simulink model "Model_TranslationEngine64"  (R2022b)
settings: Solver=FixedStepDiscrete  StartTime=0.0  StopTime=5  RelTol=1e-3  EnableMultiTasking=on
InitFcn:
  | % Initialize model
  | ModelSettings=BTConfig.GetModelSettings();
  | 
  | ModelSettings.Validate();
  | 
  | ModelInit;
  | 
  | 
  | % load library data
  | GainLibrary_data;
  | % Load saved values from partition process
  | CapturedConstMask.LoadMapFromFile(bdroot)
StartFcn:
  | % make sure all the simulated RTC requests are found
  | %RTC_SIM_OBJ.ValidateREQs();
undefined symbols (not defined in the file or in its folder): AA, BPLP, Column, NumHFRefBPF, NumHFRefLPF, NumMusicChannels, Row, VolumeMuteConfig
libraries: TuneVar x925, TOP x490, FeaturePath x111, CapturedConstLib x52
(part 15 of 34)

== system Model_TranslationEngine64/NEAR/Near1p1/VolumeMute/AnnouncementLevelDetector/ch2_level/hold_margin ==
  SetPositive : MATLAB Function  TreatAsAtomicUnit=on
  TOP : TOP/TOP  TriggerInit=[440 20 640 80]  TopName=HoldMarginDb  DataTypeOut=Inherit: Same as input  BankNumber=0  PreOverlay=false  PostOverlay=false  Role=Automatic
      settings: SourceProductName=Bose Talaria
  TranslateTrigger : TuneVar/TranslateTrigger  TriggerInit=[306 -100 344 -45]
      settings: SourceProductName=Bose Talaria
  Tune Variable : TuneVar/TuneVar  TuneName=HoldMarginDb  SpecifyMaxSize=off  VariableDim=1 (Row)  MaxSize=[1 1]  TunabilityNumber=1  MinValue=[]  MaxValue=[]  TriggerInit=[-120 22 90 78]  MaskValue=Config.DefaultAnn2LevelDetectHoldMarginDb
      settings: SourceProductName=Bose Talaria
  wires:
  TranslateTrigger/1 -> SetPositive/Trigger
  SetPositive/1(TOP) -> TOP/1
  Tune Variable/1 -> SetPositive/1(Tune)  "HoldMarginDb"

== system Model_TranslationEngine64/NEAR/Near1p1/VolumeMute/AnnouncementLevelDetector/ch2_level/hold_time ==
  TOP : TOP/TOP  TriggerInit=[475 15 725 85]  TopName=HoldTimeSamples  DataTypeOut=Inherit: Same as input  BankNumber=0  PreOverlay=false  PostOverlay=false  Role=Automatic
      settings: SourceProductName=Bose Talaria
  TranslateTrigger : TuneVar/TranslateTrigger  TriggerInit=[306 -100 344 -45]
      settings: SourceProductName=Bose Talaria
  Tune Variable : TuneVar/TuneVar  TuneName=HoldTimes  SpecifyMaxSize=off  VariableDim=1 (Row)  MaxSize=[1 1]  TunabilityNumber=1  MinValue=[]  MaxValue=[]  TriggerInit=[-100 15 150 85]  MaskValue=Config.DefaultAnn2LevelDetectHoldTimes
      settings: SourceProductName=Bose Talaria
  sec2samples : MATLAB Function  TreatAsAtomicUnit=on  mask{FrameRate=Config.FrameRate}
  wires:
  TranslateTrigger/1 -> sec2samples/Trigger
  sec2samples/1(y) -> TOP/1
  Tune Variable/1 -> sec2samples/1(u)  "HoldTimes"

== system Model_TranslationEngine64/NEAR/Near1p1/VolumeMute/AnnouncementLevelDetector/ch2_level/max_volume ==
  TOP : TOP/TOP  TriggerInit=[440 20 585 80]  TopName=MaxVolumeDb  DataTypeOut=single  BankNumber=BankNumber  PreOverlay=PreOverlay  PostOverlay=PostOverlay  Role=Automatic
      settings: SourceProductName=Bose Talaria
  TrivialTranslation : TuneVar/TrivialTranslation  TriggerInit=[300 28 350 72]
      settings: SourceProductName=Bose Talaria
  Tune Variable : TuneVar/TuneVar  TuneName=MaxVolumeDb  SpecifyMaxSize=off  VariableDim=1 (Row)  MaxSize=[1 1]  TunabilityNumber=1  MinValue=MinValue  MaxValue=MaxValue  TriggerInit=[20 25 190 75]  MaskValue=MaskValue
      settings: SourceProductName=Bose Talaria
  wires:
  Tune Variable/1 -> TrivialTranslation/1  "MaxVolumeDb"
  TrivialTranslation/1 -> TOP/1

== system Model_TranslationEngine64/NEAR/Near1p1/VolumeMute/AnnouncementLevelDetector/ch2_level/min_volume ==
  TOP : TOP/TOP  TriggerInit=[440 20 585 80]  TopName=MinVolumeDb  DataTypeOut=single  BankNumber=BankNumber  PreOverlay=PreOverlay  PostOverlay=PostOverlay  Role=Automatic
      settings: SourceProductName=Bose Talaria
  TrivialTranslation : TuneVar/TrivialTranslation  TriggerInit=[300 28 350 72]
      settings: SourceProductName=Bose Talaria
  Tune Variable : TuneVar/TuneVar  TuneName=MinVolumeDb  SpecifyMaxSize=off  VariableDim=1 (Row)  MaxSize=[1 1]  TunabilityNumber=1  MinValue=MinValue  MaxValue=MaxValue  TriggerInit=[20 25 190 75]  MaskValue=MaskValue
      settings: SourceProductName=Bose Talaria
  wires:
  Tune Variable/1 -> TrivialTranslation/1  "MinVolumeDb"
  TrivialTranslation/1 -> TOP/1

== system Model_TranslationEngine64/NEAR/Near1p1/VolumeMute/AnnouncementLevelDetector/ch2_level/slow_decay ==
  TOP : TOP/TOP  TriggerInit=[440 17 695 83]  TopName=SlowDecayDbPerSample  DataTypeOut=Inherit: Same as input  BankNumber=0  PreOverlay=false  PostOverlay=false  Role=Automatic
      settings: SourceProductName=Bose Talaria
  TranslateTrigger : TuneVar/TranslateTrigger  TriggerInit=[306 -100 344 -45]
      settings: SourceProductName=Bose Talaria
  Tune Variable : TuneVar/TuneVar  TuneName=SlowDecayDbPers  SpecifyMaxSize=off  VariableDim=1 (Row)  MaxSize=[1 1]  TunabilityNumber=1  MinValue=[]  MaxValue=[]  TriggerInit=[-100 17 155 83]  MaskValue=Config.DefaultAnn2LevelDetectSlowDecayDbPers
      settings: SourceProductName=Bose Talaria
  sec2samples : MATLAB Function  TreatAsAtomicUnit=on  mask{FrameRate=Config.FrameRate}
  wires:
  TranslateTrigger/1 -> sec2samples/Trigger
  sec2samples/1(y) -> TOP/1
  Tune Variable/1 -> sec2samples/1(u)  "SlowDecayDbPers"

== system Model_TranslationEngine64/NEAR/Near1p1/VolumeMute/AnnouncementLevelDetector/ch3_level/fast_decay ==
  TOP : TOP/TOP  TriggerInit=[415 20 675 80]  TopName=FastDecayDbPerSample  DataTypeOut=Inherit: Same as input  BankNumber=0  PreOverlay=false  PostOverlay=false  Role=Automatic
      settings: SourceProductName=Bose Talaria
  TranslateTrigger : TuneVar/TranslateTrigger  TriggerInit=[291 -100 329 -45]
      settings: SourceProductName=Bose Talaria
  Tune Variable : TuneVar/TuneVar  TuneName=FastDecayDbPers  SpecifyMaxSize=off  VariableDim=1 (Row)  MaxSize=[1 1]  TunabilityNumber=1  MinValue=[]  MaxValue=[]  TriggerInit=[-135 20 125 80]  MaskValue=Config.DefaultAnn3LevelDetectFastDecayDbPers
      settings: SourceProductName=Bose Talaria
  sec2samples : MATLAB Function  TreatAsAtomicUnit=on  mask{FrameRate=Config.FrameRate}
  wires:
  TranslateTrigger/1 -> sec2samples/Trigger
  sec2samples/1(y) -> TOP/1
  Tune Variable/1 -> sec2samples/1(u)  "FastDecayDbPers"

== system Model_TranslationEngine64/NEAR/Near1p1/VolumeMute/AnnouncementLevelDetector/ch3_level/hold_margin ==
  SetPositive : MATLAB Function  TreatAsAtomicUnit=on
  TOP : TOP/TOP  TriggerInit=[440 20 640 80]  TopName=HoldMarginDb  DataTypeOut=Inherit: Same as input  BankNumber=0  PreOverlay=false  PostOverlay=false  Role=Automatic
      settings: SourceProductName=Bose Talaria
  TranslateTrigger : TuneVar/TranslateTrigger  TriggerInit=[306 -100 344 -45]
      settings: SourceProductName=Bose Talaria
  Tune Variable : TuneVar/TuneVar  TuneName=HoldMarginDb  SpecifyMaxSize=off  VariableDim=1 (Row)  MaxSize=[1 1]  TunabilityNumber=1  MinValue=[]  MaxValue=[]  TriggerInit=[-120 22 90 78]  MaskValue=Config.DefaultAnn3LevelDetectHoldMarginDb
      settings: SourceProductName=Bose Talaria
  wires:
  Tune Variable/1 -> SetPositive/1(Tune)  "HoldMarginDb"
  SetPositive/1(TOP) -> TOP/1
  TranslateTrigger/1 -> SetPositive/Trigger

== system Model_TranslationEngine64/NEAR/Near1p1/VolumeMute/AnnouncementLevelDetector/ch3_level/hold_time ==
  TOP : TOP/TOP  TriggerInit=[495 17 755 83]  TopName=HoldTimeSamples  DataTypeOut=Inherit: Same as input  BankNumber=0  PreOverlay=false  PostOverlay=false  Role=Automatic
      settings: SourceProductName=Bose Talaria
  TranslateTrigger : TuneVar/TranslateTrigger  TriggerInit=[306 -100 344 -45]
      settings: SourceProductName=Bose Talaria
  Tune Variable : TuneVar/TuneVar  TuneName=HoldTimes  SpecifyMaxSize=off  VariableDim=1 (Row)  MaxSize=[1 1]  TunabilityNumber=1  MinValue=[]  MaxValue=[]  TriggerInit=[-115 17 145 83]  MaskValue=Config.DefaultAnn3LevelDetectHoldTimes
      settings: SourceProductName=Bose Talaria
  sec2samples : MATLAB Function  TreatAsAtomicUnit=on  mask{FrameRate=Config.FrameRate}
  wires:
  TranslateTrigger/1 -> sec2samples/Trigger
  sec2samples/1(y) -> TOP/1
  Tune Variable/1 -> sec2samples/1(u)  "HoldTimes"

== system Model_TranslationEngine64/NEAR/Near1p1/VolumeMute/AnnouncementLevelDetector/ch3_level/max_volume1 ==
  TOP : TOP/TOP  TriggerInit=[440 20 585 80]  TopName=MaxVolumeDb  DataTypeOut=single  BankNumber=BankNumber  PreOverlay=PreOverlay  PostOverlay=PostOverlay  Role=Automatic
      settings: SourceProductName=Bose Talaria
  TrivialTranslation : TuneVar/TrivialTranslation  TriggerInit=[300 28 350 72]
      settings: SourceProductName=Bose Talaria
  Tune Variable : TuneVar/TuneVar  TuneName=MaxVolumeDb  SpecifyMaxSize=off  VariableDim=1 (Row)  MaxSize=[1 1]  TunabilityNumber=1  MinValue=MinValue  MaxValue=MaxValue  TriggerInit=[20 25 190 75]  MaskValue=MaskValue
      settings: SourceProductName=Bose Talaria
  wires:
  Tune Variable/1 -> TrivialTranslation/1  "MaxVolumeDb"
  TrivialTranslation/1 -> TOP/1

== system Model_TranslationEngine64/NEAR/Near1p1/VolumeMute/AnnouncementLevelDetector/ch3_level/min_volume1 ==
  TOP : TOP/TOP  TriggerInit=[440 20 585 80]  TopName=MinVolumeDb  DataTypeOut=single  BankNumber=BankNumber  PreOverlay=PreOverlay  PostOverlay=PostOverlay  Role=Automatic
      settings: SourceProductName=Bose Talaria
  TrivialTranslation : TuneVar/TrivialTranslation  TriggerInit=[300 28 350 72]
      settings: SourceProductName=Bose Talaria
  Tune Variable : TuneVar/TuneVar  TuneName=MinVolumeDb  SpecifyMaxSize=off  VariableDim=1 (Row)  MaxSize=[1 1]  TunabilityNumber=1  MinValue=MinValue  MaxValue=MaxValue  TriggerInit=[20 25 190 75]  MaskValue=MaskValue
      settings: SourceProductName=Bose Talaria
  wires:
  Tune Variable/1 -> TrivialTranslation/1  "MinVolumeDb"
  TrivialTranslation/1 -> TOP/1

== system Model_TranslationEngine64/NEAR/Near1p1/VolumeMute/AnnouncementLevelDetector/ch3_level/slow_decay ==
  TOP : TOP/TOP  TriggerInit=[440 17 695 83]  TopName=SlowDecayDbPerSample  DataTypeOut=Inherit: Same as input  BankNumber=0  PreOverlay=false  PostOverlay=false  Role=Automatic
      settings: SourceProductName=Bose Talaria
  TranslateTrigger : TuneVar/TranslateTrigger  TriggerInit=[306 -100 344 -45]
      settings: SourceProductName=Bose Talaria
  Tune Variable : TuneVar/TuneVar  TuneName=SlowDecayDbPers  SpecifyMaxSize=off  VariableDim=1 (Row)  MaxSize=[1 1]  TunabilityNumber=1  MinValue=[]  MaxValue=[]  TriggerInit=[-115 17 140 83]  MaskValue=Config.DefaultAnn3LevelDetectSlowDecayDbPers
      settings: SourceProductName=Bose Talaria
  sec2samples : MATLAB Function  TreatAsAtomicUnit=on  mask{FrameRate=Config.FrameRate}
  wires:
  Tune Variable/1 -> sec2samples/1(u)  "SlowDecayDbPers"
  sec2samples/1(y) -> TOP/1
  TranslateTrigger/1 -> sec2samples/Trigger

== system Model_TranslationEngine64/NEAR/Near1p1/VolumeMute/AnnouncementLevelDetector/ch4_level/fast_decay ==
  TOP : TOP/TOP  TriggerInit=[415 20 675 80]  TopName=FastDecayDbPerSample  DataTypeOut=Inherit: Same as input  BankNumber=0  PreOverlay=false  PostOverlay=false  Role=Automatic
      settings: SourceProductName=Bose Talaria
  TranslateTrigger : TuneVar/TranslateTrigger  TriggerInit=[291 -100 329 -45]
      settings: SourceProductName=Bose Talaria
  Tune Variable : TuneVar/TuneVar  TuneName=FastDecayDbPers  SpecifyMaxSize=off  VariableDim=1 (Row)  MaxSize=[1 1]  TunabilityNumber=1  MinValue=[]  MaxValue=[]  TriggerInit=[-135 20 125 80]  MaskValue=Config.DefaultAnn4LevelDetectFastDecayDbPers
      settings: SourceProductName=Bose Talaria
  sec2samples : MATLAB Function  TreatAsAtomicUnit=on  mask{FrameRate=Config.FrameRate}
  wires:
  TranslateTrigger/1 -> sec2samples/Trigger
  sec2samples/1(y) -> TOP/1
  Tune Variable/1 -> sec2samples/1(u)  "FastDecayDbPers"

== system Model_TranslationEngine64/NEAR/Near1p1/VolumeMute/AnnouncementLevelDetector/ch4_level/hold_margin ==
  SetPositive : MATLAB Function  TreatAsAtomicUnit=on
  TOP : TOP/TOP  TriggerInit=[440 20 640 80]  TopName=HoldMarginDb  DataTypeOut=Inherit: Same as input  BankNumber=0  PreOverlay=false  PostOverlay=false  Role=Automatic
      settings: SourceProductName=Bose Talaria
  TranslateTrigger : TuneVar/TranslateTrigger  TriggerInit=[306 -100 344 -45]
      settings: SourceProductName=Bose Talaria
  Tune Variable : TuneVar/TuneVar  TuneName=HoldMarginDb  SpecifyMaxSize=off  VariableDim=1 (Row)  MaxSize=[1 1]  TunabilityNumber=1  MinValue=[]  MaxValue=[]  TriggerInit=[-120 22 90 78]  MaskValue=Config.DefaultAnn4LevelDetectHoldMarginDb
      settings: SourceProductName=Bose Talaria
  wires:
  Tune Variable/1 -> SetPositive/1(Tune)  "HoldMarginDb"
  SetPositive/1(TOP) -> TOP/1
  TranslateTrigger/1 -> SetPositive/Trigger

== system Model_TranslationEngine64/NEAR/Near1p1/VolumeMute/AnnouncementLevelDetector/ch4_level/hold_time ==
  TOP : TOP/TOP  TriggerInit=[495 17 755 83]  TopName=HoldTimeSamples  DataTypeOut=Inherit: Same as input  BankNumber=0  PreOverlay=false  PostOverlay=false  Role=Automatic
      settings: SourceProductName=Bose Talaria
  TranslateTrigger : TuneVar/TranslateTrigger  TriggerInit=[306 -100 344 -45]
      settings: SourceProductName=Bose Talaria
  Tune Variable : TuneVar/TuneVar  TuneName=HoldTimes  SpecifyMaxSize=off  VariableDim=1 (Row)  MaxSize=[1 1]  TunabilityNumber=1  MinValue=[]  MaxValue=[]  TriggerInit=[-115 17 145 83]  MaskValue=Config.DefaultAnn4LevelDetectHoldTimes
      settings: SourceProductName=Bose Talaria
  sec2samples : MATLAB Function  TreatAsAtomicUnit=on  mask{FrameRate=Config.FrameRate}
  wires:
  TranslateTrigger/1 -> sec2samples/Trigger
  sec2samples/1(y) -> TOP/1
  Tune Variable/1 -> sec2samples/1(u)  "HoldTimes"

== system Model_TranslationEngine64/NEAR/Near1p1/VolumeMute/AnnouncementLevelDetector/ch4_level/max_volume1 ==
  TOP : TOP/TOP  TriggerInit=[440 20 585 80]  TopName=MaxVolumeDb  DataTypeOut=single  BankNumber=BankNumber  PreOverlay=PreOverlay  PostOverlay=PostOverlay  Role=Automatic
      settings: SourceProductName=Bose Talaria
  TrivialTranslation : TuneVar/TrivialTranslation  TriggerInit=[300 28 350 72]
      settings: SourceProductName=Bose Talaria
  Tune Variable : TuneVar/TuneVar  TuneName=MaxVolumeDb  SpecifyMaxSize=off  VariableDim=1 (Row)  MaxSize=[1 1]  TunabilityNumber=1  MinValue=MinValue  MaxValue=MaxValue  TriggerInit=[20 25 190 75]  MaskValue=MaskValue
      settings: SourceProductName=Bose Talaria
  wires:
  Tune Variable/1 -> TrivialTranslation/1  "MaxVolumeDb"
  TrivialTranslation/1 -> TOP/1

== system Model_TranslationEngine64/NEAR/Near1p1/VolumeMute/AnnouncementLevelDetector/ch4_level/min_volume1 ==
  TOP : TOP/TOP  TriggerInit=[440 20 585 80]  TopName=MinVolumeDb  DataTypeOut=single  BankNumber=BankNumber  PreOverlay=PreOverlay  PostOverlay=PostOverlay  Role=Automatic
      settings: SourceProductName=Bose Talaria
  TrivialTranslation : TuneVar/TrivialTranslation  TriggerInit=[300 28 350 72]
      settings: SourceProductName=Bose Talaria
  Tune Variable : TuneVar/TuneVar  TuneName=MinVolumeDb  SpecifyMaxSize=off  VariableDim=1 (Row)  MaxSize=[1 1]  TunabilityNumber=1  MinValue=MinValue  MaxValue=MaxValue  TriggerInit=[20 25 190 75]  MaskValue=MaskValue
      settings: SourceProductName=Bose Talaria
  wires:
  Tune Variable/1 -> TrivialTranslation/1  "MinVolumeDb"
  TrivialTranslation/1 -> TOP/1

== system Model_TranslationEngine64/NEAR/Near1p1/VolumeMute/AnnouncementLevelDetector/ch4_level/slow_decay ==
  TOP : TOP/TOP  TriggerInit=[445 15 710 85]  TopName=SlowDecayDbPerSample  DataTypeOut=Inherit: Same as input  BankNumber=0  PreOverlay=false  PostOverlay=false  Role=Automatic
      settings: SourceProductName=Bose Talaria
  TranslateTrigger : TuneVar/TranslateTrigger  TriggerInit=[306 -100 344 -45]
      settings: SourceProductName=Bose Talaria
  Tune Variable : TuneVar/TuneVar  TuneName=SlowDecayDbPers  SpecifyMaxSize=off  VariableDim=1 (Row)  MaxSize=[1 1]  TunabilityNumber=1  MinValue=[]  MaxValue=[]  TriggerInit=[-130 15 135 85]  MaskValue=Config.DefaultAnn4LevelDetectSlowDecayDbPers
      settings: SourceProductName=Bose Talaria
  sec2samples : MATLAB Function  TreatAsAtomicUnit=on  mask{FrameRate=Config.FrameRate}
  wires:
  TranslateTrigger/1 -> sec2samples/Trigger
  sec2samples/1(y) -> TOP/1
  Tune Variable/1 -> sec2samples/1(u)  "SlowDecayDbPers"

== system Model_TranslationEngine64/NEAR/Near1p1/VolumeMute/VolMuteCh1/Ann1NonEntGainCalc/TuneTOP ==
  TOP : TOP/TOP  TriggerInit=[440 20 585 80]  TopName=VncThresh  DataTypeOut=single  BankNumber=BankNumber  PreOverlay=PreOverlay  PostOverlay=PostOverlay  Role=Automatic
      settings: SourceProductName=Bose Talaria
  TrivialTranslation : TuneVar/TrivialTranslation  TriggerInit=[300 28 350 72]
      settings: SourceProductName=Bose Talaria
  Tune Variable : TuneVar/TuneVar  TuneName=VncThresh  SpecifyMaxSize=off  VariableDim=1 (Row)  MaxSize=[1 1]  TunabilityNumber=1  MinValue=MinValue  MaxValue=MaxValue  TriggerInit=[20 25 190 75]  MaskValue=MaskValue
      settings: SourceProductName=Bose Talaria
  wires:
  Tune Variable/1 -> TrivialTranslation/1  "VncThresh"
  TrivialTranslation/1 -> TOP/1

== system Model_TranslationEngine64/NEAR/Near1p1/VolumeMute/VolMuteCh1/Ann1NonEntGainCalc/TuneTOP1 ==
  TOP : TOP/TOP  TriggerInit=[440 20 585 80]  TopName=VncSlope  DataTypeOut=single  BankNumber=BankNumber  PreOverlay=PreOverlay  PostOverlay=PostOverlay  Role=Automatic
      settings: SourceProductName=Bose Talaria
  TrivialTranslation : TuneVar/TrivialTranslation  TriggerInit=[300 28 350 72]
      settings: SourceProductName=Bose Talaria
  Tune Variable : TuneVar/TuneVar  TuneName=VncSlope  SpecifyMaxSize=off  VariableDim=1 (Row)  MaxSize=[1 1]  TunabilityNumber=1  MinValue=MinValue  MaxValue=MaxValue  TriggerInit=[20 25 190 75]  MaskValue=MaskValue
      settings: SourceProductName=Bose Talaria
  wires:
  Tune Variable/1 -> TrivialTranslation/1  "VncSlope"
  TrivialTranslation/1 -> TOP/1

== system Model_TranslationEngine64/NEAR/Near1p1/VolumeMute/VolMuteCh1/Ann1NonEntGainCalc/TuneTOP2 ==
  TOP : TOP/TOP  TriggerInit=[440 20 585 80]  TopName=MaxBoost  DataTypeOut=single  BankNumber=BankNumber  PreOverlay=PreOverlay  PostOverlay=PostOverlay  Role=Automatic
      settings: SourceProductName=Bose Talaria
  TrivialTranslation : TuneVar/TrivialTranslation  TriggerInit=[300 28 350 72]
      settings: SourceProductName=Bose Talaria
  Tune Variable : TuneVar/TuneVar  TuneName=MaxBoost  SpecifyMaxSize=off  VariableDim=1 (Row)  MaxSize=[1 1]  TunabilityNumber=1  MinValue=MinValue  MaxValue=MaxValue  TriggerInit=[20 25 190 75]  MaskValue=MaskValue
      settings: SourceProductName=Bose Talaria
  wires:
  Tune Variable/1 -> TrivialTranslation/1  "MaxBoost"
  TrivialTranslation/1 -> TOP/1

== system Model_TranslationEngine64/NEAR/Near1p1/VolumeMute/VolMuteCh1/Ann1NonEntGainCalc/TuneTOP3 ==
  TOP : TOP/TOP  TriggerInit=[440 20 585 80]  TopName=NoiseOverRide  DataTypeOut=single  BankNumber=BankNumber  PreOverlay=PreOverlay  PostOverlay=PostOverlay  Role=Automatic
      settings: SourceProductName=Bose Talaria
  TrivialTranslation : TuneVar/TrivialTranslation  TriggerInit=[300 28 350 72]
      settings: SourceProductName=Bose Talaria
  Tune Variable : TuneVar/TuneVar  TuneName=NoiseOverRide  SpecifyMaxSize=off  VariableDim=1 (Row)  MaxSize=[1 1]  TunabilityNumber=1  MinValue=MinValue  MaxValue=MaxValue  TriggerInit=[20 25 190 75]  MaskValue=MaskValue
      settings: SourceProductName=Bose Talaria
  wires:
  Tune Variable/1 -> TrivialTranslation/1  "NoiseOverRide"
  TrivialTranslation/1 -> TOP/1

== system Model_TranslationEngine64/NEAR/Near1p1/VolumeMute/VolMuteCh1/Ann1NonEntGainCalc/TuneTOP4 ==
  TOP : TOP/TOP  TriggerInit=[440 20 585 80]  TopName=NoiseOverRideFlag  DataTypeOut=single  BankNumber=BankNumber  PreOverlay=PreOverlay  PostOverlay=PostOverlay  Role=Automatic
      settings: SourceProductName=Bose Talaria
  TrivialTranslation : TuneVar/TrivialTranslation  TriggerInit=[300 28 350 72]
      settings: SourceProductName=Bose Talaria
  Tune Variable : TuneVar/TuneVar  TuneName=NoiseOverRideFlag  SpecifyMaxSize=off  VariableDim=1 (Row)  MaxSize=[1 1]  TunabilityNumber=1  MinValue=MinValue  MaxValue=MaxValue  TriggerInit=[20 25 190 75]  MaskValue=MaskValue
      settings: SourceProductName=Bose Talaria
  wires:
  Tune Variable/1 -> TrivialTranslation/1  "NoiseOverRideFlag"
  TrivialTranslation/1 -> TOP/1

== system Model_TranslationEngine64/NEAR/Near1p1/VolumeMute/VolMuteCh1/Ann1NonEntGainCalc/TuneTOP5 ==
  TOP : TOP/TOP  TriggerInit=[440 20 585 80]  TopName=BoostOverRide  DataTypeOut=single  BankNumber=BankNumber  PreOverlay=PreOverlay  PostOverlay=PostOverlay  Role=Automatic
      settings: SourceProductName=Bose Talaria
  TrivialTranslation : TuneVar/TrivialTranslation  TriggerInit=[300 28 350 72]
      settings: SourceProductName=Bose Talaria
  Tune Variable : TuneVar/TuneVar  TuneName=BoostOverRide  SpecifyMaxSize=off  VariableDim=1 (Row)  MaxSize=[1 1]  TunabilityNumber=1  MinValue=MinValue  MaxValue=MaxValue  TriggerInit=[20 25 190 75]  MaskValue=MaskValue
      settings: SourceProductName=Bose Talaria
  wires:
  Tune Variable/1 -> TrivialTranslation/1  "BoostOverRide"
  TrivialTranslation/1 -> TOP/1

== system Model_TranslationEngine64/NEAR/Near1p1/VolumeMute/VolMuteCh1/Ann1NonEntGainCalc/TuneTOP6 ==
  TOP : TOP/TOP  TriggerInit=[440 20 585 80]  TopName=BoostOverRideFlag  DataTypeOut=single  BankNumber=BankNumber  PreOverlay=PreOverlay  PostOverlay=PostOverlay  Role=Automatic
      settings: SourceProductName=Bose Talaria
  TrivialTranslation : TuneVar/TrivialTranslation  TriggerInit=[300 28 350 72]
      settings: SourceProductName=Bose Talaria
  Tune Variable : TuneVar/TuneVar  TuneName=BoostOverRideFlag  SpecifyMaxSize=off  VariableDim=1 (Row)  MaxSize=[1 1]  TunabilityNumber=1  MinValue=MinValue  MaxValue=MaxValue  TriggerInit=[20 25 190 75]  MaskValue=MaskValue
      settings: SourceProductName=Bose Talaria
  wires:
  Tune Variable/1 -> TrivialTranslation/1  "BoostOverRideFlag"
  TrivialTranslation/1 -> TOP/1

== system Model_TranslationEngine64/NEAR/Near1p1/VolumeMute/VolMuteCh1/Ann1NonEntGainCalc/TuneTOP7 ==
  TOP : TOP/TOP  TriggerInit=[440 20 585 80]  TopName=VncEnableTuneVar  DataTypeOut=single  BankNumber=BankNumber  PreOverlay=PreOverlay  PostOverlay=PostOverlay  Role=Automatic
      settings: SourceProductName=Bose Talaria
  TrivialTranslation : TuneVar/TrivialTranslation  TriggerInit=[300 28 350 72]
      settings: SourceProductName=Bose Talaria
  Tune Variable : TuneVar/TuneVar  TuneName=VncEnableTuneVar  SpecifyMaxSize=off  VariableDim=1 (Row)  MaxSize=[1 1]  TunabilityNumber=1  MinValue=MinValue  MaxValue=MaxValue  TriggerInit=[20 25 190 75]  MaskValue=MaskValue
      settings: SourceProductName=Bose Talaria
  wires:
  Tune Variable/1 -> TrivialTranslation/1  "VncEnableTuneVar"
  TrivialTranslation/1 -> TOP/1

== system Model_TranslationEngine64/NEAR/Near1p1/VolumeMute/VolMuteCh1/Ann1NonEntGainCalc/TuneTOP8 ==
  TranslateTrigger : TuneVar/TranslateTrigger  TriggerInit=[306 -100 344 -45]
      settings: SourceProductName=Bose Talaria
  den : TOP/TOP  TriggerInit=[450 90 595 150]  TopName=Den  DataTypeOut=single  BankNumber=0  PreOverlay=false  PostOverlay=false  Role=Automatic
      settings: SourceProductName=Bose Talaria
  num : TOP/TOP  TriggerInit=[450 -45 595 15]  TopName=Num  DataTypeOut=single  BankNumber=0  PreOverlay=false  PostOverlay=false  Role=Automatic
      settings: SourceProductName=Bose Talaria
  translation : MATLAB Function  TreatAsAtomicUnit=on  mask{L=Config.FrameSize, Fd=Config.Fd}
  tuneVARTau : TuneVar/TuneVar  TuneName=Tau  SpecifyMaxSize=off  VariableDim=1 (Row)  MaxSize=[1 1]  TunabilityNumber=1  MinValue=[]  MaxValue=[]  TriggerInit=[-70 25 100 75]  MaskValue=Config.DefaultTau
      settings: SourceProductName=Bose Talaria
  wires:
  tuneVARTau/1 -> translation/1(tau)  "Tau"
  TranslateTrigger/1 -> translation/Trigger
  translation/2(Den) -> den/1
  translation/1(Num) -> num/1

== system Model_TranslationEngine64/NEAR/Near1p1/VolumeMute/VolMuteCh1/Ann1NonEntGainCalc/vncSignal ==
  TuneTOP : Subsystem  mask(Talaria Trivial Tune TOP){TriggerInit=[50 -8 220 48], TopName=MinVncSignal, TuneName=MinVncSignal, DataTypeOut=single, MaskValue=Config.DefaultMinVncSignal, TunabilityNumber=1, MinValue=[], MaxValue=[], BankNumber=0, PreOverlay=false, PostOverlay=false, UseSameName=on}
      mask prompts: TriggerInit "Hidden: MoveFcn redraw"; TopName "Name:"; TuneName "Name of TuneVar:"; DataTypeOut "Data type:"; MaskValue "Default Value:"; TunabilityNumber "Tunability:"; MinValue "Min Value:"; MaxValue "Max Value:"; BankNumber "Target memory bank number:"; PreOverlay "Requires pre-overlay action:"; PostOverlay "Requires post-overlay action:"; UseSameName "Use same name for tune variable and TOP"
      mask help: The TuneTOP block encapsultes a Target Overlay Parameter, a Tune Variable, and a Trivial Translation between them.
      mask init:
      | [ok,activeTopPath,activeTunePath] = TuneTOP_Mask.Init(gcbh);
      settings: MoveFcn=TuneTOP_Mask.CB_TriggerInit(gcbh);
      mask Callback TriggerInit: TuneTOP_Mask.CB_TriggerInit(gcbh);
      mask TypeOptions TopName: TOP/TopName
      mask TypeOptions TuneName: Tune Variable/TuneName
      mask TypeOptions DataTypeOut: TOP/DataTypeOut
      mask TypeOptions MaskValue: Tune Variable/MaskValue
      mask TypeOptions TunabilityNumber: Tune Variable/TunabilityNumber
      mask Callback TunabilityNumber: TuneVarMask.CB_TunabilityNumber(gcbh);
      mask TypeOptions MinValue: Tune Variable/MinValue
      mask TypeOptions MaxValue: Tune Variable/MaxValue
      mask TypeOptions BankNumber: TOP/BankNumber
      mask TypeOptions PreOverlay: TOP/PreOverlay
      mask TypeOptions PostOverlay: TOP/PostOverlay
      mask Callback UseSameName: TuneTOP_Mask.CB_UseSameName(gcbh);
      mask DialogControl toolPanel Prompt: Tuning Tool Hints
      mask DialogControl DescriptionGroup Prompt: Description
      mask DialogControl EditDescription Prompt: Edit Description
      mask DialogControl EditDescription Callback: TuneTOP_Mask.CB_EditDescription(gcbh);
      mask DialogControl TunabilityText Prompt: Easy: Changes nearly every tuning.
      mask DialogControl AdvancedPanel Prompt: Advanced
      mask DialogControl ConvertToFullTranslation Prompt: Irreversible conversion to full translation
      mask DialogControl ConvertToFullTranslation Callback: TuneTOP_Mask.CB_ConvertToFullTranslation(gcbh);
      mask DialogControl ErrorContainer Prompt: Error Messages
      mask Display:
      | % retrieve icon definition
      | [path,w,h] = TuneTOP_Mask.Icon();
      | 
      | % retrieve the block's pixel size
      | pos = get(gcbh,'position');
      | bw = pos(3) - pos(1);
      | bh = pos(4) - pos(2);
      | 
      | % draw centered icon
      | xAdj = bw/2 - w/2 + 5;
      | yAdj = bh/2 - h/2 + 4;
      | for i=1:length(path)
      | 	patch(path(i).x+xAdj, path(i).y+yAdj, path(i).rgb);
      | end
      | 
      | % show the top name or an X
      | if (exist('ok','var') && ok)
      | 	text(bw*0.5, bh*0.2, activeTopPath, 'horizontalAlignment', 'center');
      | 	patch(0,0,[1 1 1]);
      | 	patch(bw,bh,[1 1 1]);
      | else
      | 	tx=bw*0.03;
      | 	ty=bh*0.03;
      | 	patch([0 tx bw bw-tx], [ty 0 bh-ty bh], [1 0 0]);
      | 	patch([0 bw-tx bw tx], [bh-ty 0 ty bh], [1 0 0]);
      | end
  TuneTOP1 : Subsystem  mask(Talaria Trivial Tune TOP){TriggerInit=[40 142 210 198], TopName=MaxSpl, TuneName=MaxSpl, DataTypeOut=single, MaskValue=Config.DefaultMaxSpl, TunabilityNumber=1, MinValue=[], MaxValue=[], BankNumber=0, PreOverlay=false, PostOverlay=false, UseSameName=on}
      mask prompts: TriggerInit "Hidden: MoveFcn redraw"; TopName "Name:"; TuneName "Name of TuneVar:"; DataTypeOut "Data type:"; MaskValue "Default Value:"; TunabilityNumber "Tunability:"; MinValue "Min Value:"; MaxValue "Max Value:"; BankNumber "Target memory bank number:"; PreOverlay "Requires pre-overlay action:"; PostOverlay "Requires post-overlay action:"; UseSameName "Use same name for tune variable and TOP"
      mask help: The TuneTOP block encapsultes a Target Overlay Parameter, a Tune Variable, and a Trivial Translation between them.
      mask init:
      | [ok,activeTopPath,activeTunePath] = TuneTOP_Mask.Init(gcbh);
      settings: MoveFcn=TuneTOP_Mask.CB_TriggerInit(gcbh);
      mask Callback TriggerInit: TuneTOP_Mask.CB_TriggerInit(gcbh);
      mask TypeOptions TopName: TOP/TopName
      mask TypeOptions TuneName: Tune Variable/TuneName
      mask TypeOptions DataTypeOut: TOP/DataTypeOut
      mask TypeOptions MaskValue: Tune Variable/MaskValue
      mask TypeOptions TunabilityNumber: Tune Variable/TunabilityNumber
      mask Callback TunabilityNumber: TuneVarMask.CB_TunabilityNumber(gcbh);
      mask TypeOptions MinValue: Tune Variable/MinValue
      mask TypeOptions MaxValue: Tune Variable/MaxValue
      mask TypeOptions BankNumber: TOP/BankNumber
      mask TypeOptions PreOverlay: TOP/PreOverlay
      mask TypeOptions PostOverlay: TOP/PostOverlay
      mask Callback UseSameName: TuneTOP_Mask.CB_UseSameName(gcbh);
      mask DialogControl toolPanel Prompt: Tuning Tool Hints
      mask DialogControl DescriptionGroup Prompt: Description
      mask DialogControl EditDescription Prompt: Edit Description
      mask DialogControl EditDescription Callback: TuneTOP_Mask.CB_EditDescription(gcbh);
      mask DialogControl TunabilityText Prompt: Easy: Changes nearly every tuning.
      mask DialogControl AdvancedPanel Prompt: Advanced
      mask DialogControl ConvertToFullTranslation Prompt: Irreversible conversion to full translation
      mask DialogControl ConvertToFullTranslation Callback: TuneTOP_Mask.CB_ConvertToFullTranslation(gcbh);
      mask DialogControl ErrorContainer Prompt: Error Messages
      mask Display:
      | % retrieve icon definition
      | [path,w,h] = TuneTOP_Mask.Icon();
      | 
      | % retrieve the block's pixel size
      | pos = get(gcbh,'position');
      | bw = pos(3) - pos(1);
      | bh = pos(4) - pos(2);
      | 
      | % draw centered icon
      | xAdj = bw/2 - w/2 + 5;
      | yAdj = bh/2 - h/2 + 4;
      | for i=1:length(path)
      | 	patch(path(i).x+xAdj, path(i).y+yAdj, path(i).rgb);
      | end
      | 
      | % show the top name or an X
      | if (exist('ok','var') && ok)
      | 	text(bw*0.5, bh*0.2, activeTopPath, 'horizontalAlignment', 'center');
      | 	patch(0,0,[1 1 1]);
      | 	patch(bw,bh,[1 1 1]);
      | else
      | 	tx=bw*0.03;
      | 	ty=bh*0.03;
      | 	patch([0 tx bw bw-tx], [ty 0 bh-ty bh], [1 0 0]);
      | 	patch([0 bw-tx bw tx], [bh-ty 0 ty bh], [1 0 0]);
      | end

== system Model_TranslationEngine64/NEAR/Near1p1/VolumeMute/VolMuteCh1/Ann1NonEntVncApplied/nonentVNCApplied_subsystem ==
  TuneTOP : Subsystem

== system Model_TranslationEngine64/NEAR/Near1p1/VolumeMute/VolMuteCh1/Mute/MuteControl ==
  FeaturePath : FeaturePath/FeaturePath  FeatureName=Ann1Mute  IsGroup=off  GroupNumber=-1  IsModule=off  TriggerInit=[180 39 295 146]
      settings: SourceProductName=Bose Talaria
  TuneVarRampTime : Subsystem  Description=|  mask(Talaria Trivial Tune TOP){TriggerInit=[295 232 465 288], TopName=RampTime, TuneName=RampTime, DataTypeOut=single, MaskValue=Config.DefaultRampTimeMsec, TunabilityNumber=1, MinValue=1, MaxValue=100000, BankNumber=0, PreOverlay=false, PostOverlay=false, UseSameName=on}
      | Specifies the default value of ramp time for the Mute or Unmute operation.
      | Used only when the RTC message does not contain either ramp rate or ramp time.
      mask prompts: TriggerInit "Hidden: MoveFcn redraw"; TopName "Name:"; TuneName "Name of TuneVar:"; DataTypeOut "Data type:"; MaskValue "Default Value:"; TunabilityNumber "Tunability:"; MinValue "Min Value:"; MaxValue "Max Value:"; BankNumber "Target memory bank number:"; PreOverlay "Requires pre-overlay action:"; PostOverlay "Requires post-overlay action:"; UseSameName "Use same name for tune variable and TOP"
      mask help: The TuneTOP block encapsultes a Target Overlay Parameter, a Tune Variable, and a Trivial Translation between them.
      mask init:
      | [ok,activeTopPath,activeTunePath] = TuneTOP_Mask.Init(gcbh);
      settings: MoveFcn=TuneTOP_Mask.CB_TriggerInit(gcbh);
      mask Callback TriggerInit: TuneTOP_Mask.CB_TriggerInit(gcbh);
      mask TypeOptions TopName: TOP/TopName
      mask TypeOptions TuneName: Tune Variable/TuneName
      mask TypeOptions DataTypeOut: TOP/DataTypeOut
      mask TypeOptions MaskValue: Tune Variable/MaskValue
      mask TypeOptions TunabilityNumber: Tune Variable/TunabilityNumber
      mask Callback TunabilityNumber: TuneVarMask.CB_TunabilityNumber(gcbh);
      mask TypeOptions MinValue: Tune Variable/MinValue
      mask TypeOptions MaxValue: Tune Variable/MaxValue
      mask TypeOptions BankNumber: TOP/BankNumber
      mask TypeOptions PreOverlay: TOP/PreOverlay
      mask TypeOptions PostOverlay: TOP/PostOverlay
      mask Callback UseSameName: TuneTOP_Mask.CB_UseSameName(gcbh);
      mask DialogControl toolPanel Prompt: Tuning Tool Hints
      mask DialogControl DescriptionGroup Prompt: Description
      mask DialogControl EditDescription Prompt: Edit Description
      mask DialogControl EditDescription Callback: TuneTOP_Mask.CB_EditDescription(gcbh);
      mask DialogControl TunabilityText Prompt: Easy: Changes nearly every tuning.
      mask DialogControl AdvancedPanel Prompt: Advanced
      mask DialogControl ConvertToFullTranslation Prompt: Irreversible conversion to full translation
      mask DialogControl ConvertToFullTranslation Callback: TuneTOP_Mask.CB_ConvertToFullTranslation(gcbh);
      mask DialogControl ErrorContainer Prompt: Error Messages
      mask Display:
      | % retrieve icon definition
      | [path,w,h] = TuneTOP_Mask.Icon();
      | 
      | % retrieve the block's pixel size
      | pos = get(gcbh,'position');
      | bw = pos(3) - pos(1);
      | bh = pos(4) - pos(2);
      | 
      | % draw centered icon
      | xAdj = bw/2 - w/2 + 5;
      | yAdj = bh/2 - h/2 + 4;
      | for i=1:length(path)
      | 	patch(path(i).x+xAdj, path(i).y+yAdj, path(i).rgb);
      | end
      | 
      | % show the top name or an X
      | if (exist('ok','var') && ok)
      | 	text(bw*0.5, bh*0.2, activeTopPath, 'horizontalAlignment', 'center');
      | 	patch(0,0,[1 1 1]);
      | 	patch(bw,bh,[1 1 1]);
      | else
      | 	tx=bw*0.03;
      | 	ty=bh*0.03;
      | 	patch([0 tx bw bw-tx], [ty 0 bh-ty bh], [1 0 0]);
      | 	patch([0 bw-tx bw tx], [bh-ty 0 ty bh], [1 0 0]);
      | end

== system Model_TranslationEngine64/NEAR/Near1p1/VolumeMute/VolMuteCh1/Volume/TuneVarRampRate ==
  TOP : TOP/TOP  TriggerInit=[440 20 585 80]  TopName=RampRate  DataTypeOut=single  BankNumber=BankNumber  PreOverlay=PreOverlay  PostOverlay=PostOverlay  Role=Automatic
      settings: SourceProductName=Bose Talaria
  TrivialTranslation : TuneVar/TrivialTranslation  TriggerInit=[300 28 350 72]
      settings: SourceProductName=Bose Talaria
  Tune Variable : TuneVar/TuneVar  TuneName=RampRate  SpecifyMaxSize=off  VariableDim=1 (Row)  MaxSize=[1 1]  TunabilityNumber=2  MinValue=MinValue  MaxValue=MaxValue  TriggerInit=[20 25 190 75]  MaskValue=MaskValue
      settings: SourceProductName=Bose Talaria
  wires:
  Tune Variable/1 -> TrivialTranslation/1  "RampRate"
  TrivialTranslation/1 -> TOP/1

== system Model_TranslationEngine64/NEAR/Near1p1/VolumeMute/VolMuteCh1/Volume/TuneVarRampTime ==
  TOP : TOP/TOP  TriggerInit=[440 20 585 80]  TopName=RampTime  DataTypeOut=single  BankNumber=BankNumber  PreOverlay=PreOverlay  PostOverlay=PostOverlay  Role=Automatic
      settings: SourceProductName=Bose Talaria
  TrivialTranslation : TuneVar/TrivialTranslation  TriggerInit=[300 28 350 72]
      settings: SourceProductName=Bose Talaria
  Tune Variable : TuneVar/TuneVar  TuneName=RampTime  SpecifyMaxSize=off  VariableDim=1 (Row)  MaxSize=[1 1]  TunabilityNumber=1  MinValue=MinValue  MaxValue=MaxValue  TriggerInit=[20 25 190 75]  MaskValue=MaskValue
      settings: SourceProductName=Bose Talaria
  wires:
  Tune Variable/1 -> TrivialTranslation/1  "RampTime"
  TrivialTranslation/1 -> TOP/1

== system Model_TranslationEngine64/NEAR/Near1p1/VolumeMute/VolMuteCh2/Ann2NonEntGainCalc/TuneTOP ==
  TOP : TOP/TOP  TriggerInit=[440 20 585 80]  TopName=VncThresh  DataTypeOut=single  BankNumber=BankNumber  PreOverlay=PreOverlay  PostOverlay=PostOverlay  Role=Automatic
      settings: SourceProductName=Bose Talaria
  TrivialTranslation : TuneVar/TrivialTranslation  TriggerInit=[300 28 350 72]
      settings: SourceProductName=Bose Talaria
  Tune Variable : TuneVar/TuneVar  TuneName=VncThresh  SpecifyMaxSize=off  VariableDim=1 (Row)  MaxSize=[1 1]  TunabilityNumber=1  MinValue=MinValue  MaxValue=MaxValue  TriggerInit=[20 25 190 75]  MaskValue=MaskValue
      settings: SourceProductName=Bose Talaria
  wires:
  Tune Variable/1 -> TrivialTranslation/1  "VncThresh"
  TrivialTranslation/1 -> TOP/1

== system Model_TranslationEngine64/NEAR/Near1p1/VolumeMute/VolMuteCh2/Ann2NonEntGainCalc/TuneTOP1 ==
  TOP : TOP/TOP  TriggerInit=[440 20 585 80]  TopName=VncSlope  DataTypeOut=single  BankNumber=BankNumber  PreOverlay=PreOverlay  PostOverlay=PostOverlay  Role=Automatic
      settings: SourceProductName=Bose Talaria
  TrivialTranslation : TuneVar/TrivialTranslation  TriggerInit=[300 28 350 72]
      settings: SourceProductName=Bose Talaria
  Tune Variable : TuneVar/TuneVar  TuneName=VncSlope  SpecifyMaxSize=off  VariableDim=1 (Row)  MaxSize=[1 1]  TunabilityNumber=1  MinValue=MinValue  MaxValue=MaxValue  TriggerInit=[20 25 190 75]  MaskValue=MaskValue
      settings: SourceProductName=Bose Talaria
  wires:
  Tune Variable/1 -> TrivialTranslation/1  "VncSlope"
  TrivialTranslation/1 -> TOP/1

== system Model_TranslationEngine64/NEAR/Near1p1/VolumeMute/VolMuteCh2/Ann2NonEntGainCalc/TuneTOP2 ==
  TOP : TOP/TOP  TriggerInit=[440 20 585 80]  TopName=MaxBoost  DataTypeOut=single  BankNumber=BankNumber  PreOverlay=PreOverlay  PostOverlay=PostOverlay  Role=Automatic
      settings: SourceProductName=Bose Talaria
  TrivialTranslation : TuneVar/TrivialTranslation  TriggerInit=[300 28 350 72]
      settings: SourceProductName=Bose Talaria
  Tune Variable : TuneVar/TuneVar  TuneName=MaxBoost  SpecifyMaxSize=off  VariableDim=1 (Row)  MaxSize=[1 1]  TunabilityNumber=1  MinValue=MinValue  MaxValue=MaxValue  TriggerInit=[20 25 190 75]  MaskValue=MaskValue
      settings: SourceProductName=Bose Talaria
  wires:
  Tune Variable/1 -> TrivialTranslation/1  "MaxBoost"
  TrivialTranslation/1 -> TOP/1

== system Model_TranslationEngine64/NEAR/Near1p1/VolumeMute/VolMuteCh2/Ann2NonEntGainCalc/TuneTOP3 ==
  TOP : TOP/TOP  TriggerInit=[440 20 585 80]  TopName=NoiseOverRide  DataTypeOut=single  BankNumber=BankNumber  PreOverlay=PreOverlay  PostOverlay=PostOverlay  Role=Automatic
      settings: SourceProductName=Bose Talaria
  TrivialTranslation : TuneVar/TrivialTranslation  TriggerInit=[300 28 350 72]
      settings: SourceProductName=Bose Talaria
  Tune Variable : TuneVar/TuneVar  TuneName=NoiseOverRide  SpecifyMaxSize=off  VariableDim=1 (Row)  MaxSize=[1 1]  TunabilityNumber=1  MinValue=MinValue  MaxValue=MaxValue  TriggerInit=[20 25 190 75]  MaskValue=MaskValue
      settings: SourceProductName=Bose Talaria
  wires:
  Tune Variable/1 -> TrivialTranslation/1  "NoiseOverRide"
  TrivialTranslation/1 -> TOP/1

== system Model_TranslationEngine64/NEAR/Near1p1/VolumeMute/VolMuteCh2/Ann2NonEntGainCalc/TuneTOP4 ==
  TOP : TOP/TOP  TriggerInit=[440 20 585 80]  TopName=NoiseOverRideFlag  DataTypeOut=single  BankNumber=BankNumber  PreOverlay=PreOverlay  PostOverlay=PostOverlay  Role=Automatic
      settings: SourceProductName=Bose Talaria
  TrivialTranslation : TuneVar/TrivialTranslation  TriggerInit=[300 28 350 72]
      settings: SourceProductName=Bose Talaria
  Tune Variable : TuneVar/TuneVar  TuneName=NoiseOverRideFlag  SpecifyMaxSize=off  VariableDim=1 (Row)  MaxSize=[1 1]  TunabilityNumber=1  MinValue=MinValue  MaxValue=MaxValue  TriggerInit=[20 25 190 75]  MaskValue=MaskValue
      settings: SourceProductName=Bose Talaria
  wires:
  Tune Variable/1 -> TrivialTranslation/1  "NoiseOverRideFlag"
  TrivialTranslation/1 -> TOP/1

== system Model_TranslationEngine64/NEAR/Near1p1/VolumeMute/VolMuteCh2/Ann2NonEntGainCalc/TuneTOP5 ==
  TOP : TOP/TOP  TriggerInit=[440 20 585 80]  TopName=BoostOverRide  DataTypeOut=single  BankNumber=BankNumber  PreOverlay=PreOverlay  PostOverlay=PostOverlay  Role=Automatic
      settings: SourceProductName=Bose Talaria
  TrivialTranslation : TuneVar/TrivialTranslation  TriggerInit=[300 28 350 72]
      settings: SourceProductName=Bose Talaria
  Tune Variable : TuneVar/TuneVar  TuneName=BoostOverRide  SpecifyMaxSize=off  VariableDim=1 (Row)  MaxSize=[1 1]  TunabilityNumber=1  MinValue=MinValue  MaxValue=MaxValue  TriggerInit=[20 25 190 75]  MaskValue=MaskValue
      settings: SourceProductName=Bose Talaria
  wires:
  Tune Variable/1 -> TrivialTranslation/1  "BoostOverRide"
  TrivialTranslation/1 -> TOP/1

== system Model_TranslationEngine64/NEAR/Near1p1/VolumeMute/VolMuteCh2/Ann2NonEntGainCalc/TuneTOP6 ==
  TOP : TOP/TOP  TriggerInit=[440 20 585 80]  TopName=BoostOverRideFlag  DataTypeOut=single  BankNumber=BankNumber  PreOverlay=PreOverlay  PostOverlay=PostOverlay  Role=Automatic
      settings: SourceProductName=Bose Talaria
  TrivialTranslation : TuneVar/TrivialTranslation  TriggerInit=[300 28 350 72]
      settings: SourceProductName=Bose Talaria
  Tune Variable : TuneVar/TuneVar  TuneName=BoostOverRideFlag  SpecifyMaxSize=off  VariableDim=1 (Row)  MaxSize=[1 1]  TunabilityNumber=1  MinValue=MinValue  MaxValue=MaxValue  TriggerInit=[20 25 190 75]  MaskValue=MaskValue
      settings: SourceProductName=Bose Talaria
  wires:
  Tune Variable/1 -> TrivialTranslation/1  "BoostOverRideFlag"
  TrivialTranslation/1 -> TOP/1

== system Model_TranslationEngine64/NEAR/Near1p1/VolumeMute/VolMuteCh2/Ann2NonEntGainCalc/TuneTOP7 ==
  TOP : TOP/TOP  TriggerInit=[440 20 585 80]  TopName=VncEnableTuneVar  DataTypeOut=single  BankNumber=BankNumber  PreOverlay=PreOverlay  PostOverlay=PostOverlay  Role=Automatic
      settings: SourceProductName=Bose Talaria
  TrivialTranslation : TuneVar/TrivialTranslation  TriggerInit=[300 28 350 72]
      settings: SourceProductName=Bose Talaria
  Tune Variable : TuneVar/TuneVar  TuneName=VncEnableTuneVar  SpecifyMaxSize=off  VariableDim=1 (Row)  MaxSize=[1 1]  TunabilityNumber=1  MinValue=MinValue  MaxValue=MaxValue  TriggerInit=[20 25 190 75]  MaskValue=MaskValue
      settings: SourceProductName=Bose Talaria
  wires:
  Tune Variable/1 -> TrivialTranslation/1  "VncEnableTuneVar"
  TrivialTranslation/1 -> TOP/1

== system Model_TranslationEngine64/NEAR/Near1p1/VolumeMute/VolMuteCh2/Ann2NonEntGainCalc/TuneTOP8 ==
  TranslateTrigger : TuneVar/TranslateTrigger  TriggerInit=[306 -100 344 -45]
      settings: SourceProductName=Bose Talaria
  den : TOP/TOP  TriggerInit=[450 90 595 150]  TopName=Den  DataTypeOut=single  BankNumber=0  PreOverlay=false  PostOverlay=false  Role=Automatic
      settings: SourceProductName=Bose Talaria
  num : TOP/TOP  TriggerInit=[450 -45 595 15]  TopName=Num  DataTypeOut=single  BankNumber=0  PreOverlay=false  PostOverlay=false  Role=Automatic
      settings: SourceProductName=Bose Talaria
  translation : MATLAB Function  TreatAsAtomicUnit=on  mask{L=Config.FrameSize, Fd=Config.Fd}
  tuneVARTau : TuneVar/TuneVar  TuneName=Tau  SpecifyMaxSize=off  VariableDim=1 (Row)  MaxSize=[1 1]  TunabilityNumber=1  MinValue=[]  MaxValue=[]  TriggerInit=[-70 25 100 75]  MaskValue=Config.DefaultTau
      settings: SourceProductName=Bose Talaria
  wires:
  tuneVARTau/1 -> translation/1(tau)  "Tau"
  TranslateTrigger/1 -> translation/Trigger
  translation/2(Den) -> den/1
  translation/1(Num) -> num/1

== system Model_TranslationEngine64/NEAR/Near1p1/VolumeMute/VolMuteCh2/Ann2NonEntGainCalc/vncSignal ==
  TuneTOP : Subsystem  mask(Talaria Trivial Tune TOP){TriggerInit=[50 -8 220 48], TopName=MinVncSignal, TuneName=MinVncSignal, DataTypeOut=single, MaskValue=Config.DefaultMinVncSignal, TunabilityNumber=1, MinValue=[], MaxValue=[], BankNumber=0, PreOverlay=false, PostOverlay=false, UseSameName=on}
      mask prompts: TriggerInit "Hidden: MoveFcn redraw"; TopName "Name:"; TuneName "Name of TuneVar:"; DataTypeOut "Data type:"; MaskValue "Default Value:"; TunabilityNumber "Tunability:"; MinValue "Min Value:"; MaxValue "Max Value:"; BankNumber "Target memory bank number:"; PreOverlay "Requires pre-overlay action:"; PostOverlay "Requires post-overlay action:"; UseSameName "Use same name for tune variable and TOP"
      mask help: The TuneTOP block encapsultes a Target Overlay Parameter, a Tune Variable, and a Trivial Translation between them.
      mask init:
      | [ok,activeTopPath,activeTunePath] = TuneTOP_Mask.Init(gcbh);
      settings: MoveFcn=TuneTOP_Mask.CB_TriggerInit(gcbh);
      mask Callback TriggerInit: TuneTOP_Mask.CB_TriggerInit(gcbh);
      mask TypeOptions TopName: TOP/TopName
      mask TypeOptions TuneName: Tune Variable/TuneName
      mask TypeOptions DataTypeOut: TOP/DataTypeOut
      mask TypeOptions MaskValue: Tune Variable/MaskValue
      mask TypeOptions TunabilityNumber: Tune Variable/TunabilityNumber
      mask Callback TunabilityNumber: TuneVarMask.CB_TunabilityNumber(gcbh);
      mask TypeOptions MinValue: Tune Variable/MinValue
      mask TypeOptions MaxValue: Tune Variable/MaxValue
      mask TypeOptions BankNumber: TOP/BankNumber
      mask TypeOptions PreOverlay: TOP/PreOverlay
      mask TypeOptions PostOverlay: TOP/PostOverlay
      mask Callback UseSameName: TuneTOP_Mask.CB_UseSameName(gcbh);
      mask DialogControl toolPanel Prompt: Tuning Tool Hints
      mask DialogControl DescriptionGroup Prompt: Description
      mask DialogControl EditDescription Prompt: Edit Description
      mask DialogControl EditDescription Callback: TuneTOP_Mask.CB_EditDescription(gcbh);
      mask DialogControl TunabilityText Prompt: Easy: Changes nearly every tuning.
      mask DialogControl AdvancedPanel Prompt: Advanced
      mask DialogControl ConvertToFullTranslation Prompt: Irreversible conversion to full translation
      mask DialogControl ConvertToFullTranslation Callback: TuneTOP_Mask.CB_ConvertToFullTranslation(gcbh);
      mask DialogControl ErrorContainer Prompt: Error Messages
      mask Display:
      | % retrieve icon definition
      | [path,w,h] = TuneTOP_Mask.Icon();
      | 
      | % retrieve the block's pixel size
      | pos = get(gcbh,'position');
      | bw = pos(3) - pos(1);
      | bh = pos(4) - pos(2);
      | 
      | % draw centered icon
      | xAdj = bw/2 - w/2 + 5;
      | yAdj = bh/2 - h/2 + 4;
      | for i=1:length(path)
      | 	patch(path(i).x+xAdj, path(i).y+yAdj, path(i).rgb);
      | end
      | 
      | % show the top name or an X
      | if (exist('ok','var') && ok)
      | 	text(bw*0.5, bh*0.2, activeTopPath, 'horizontalAlignment', 'center');
      | 	patch(0,0,[1 1 1]);
      | 	patch(bw,bh,[1 1 1]);
      | else
      | 	tx=bw*0.03;
      | 	ty=bh*0.03;
      | 	patch([0 tx bw bw-tx], [ty 0 bh-ty bh], [1 0 0]);
      | 	patch([0 bw-tx bw tx], [bh-ty 0 ty bh], [1 0 0]);
      | end
  TuneTOP1 : Subsystem  mask(Talaria Trivial Tune TOP){TriggerInit=[40 142 210 198], TopName=MaxSpl, TuneName=MaxSpl, DataTypeOut=single, MaskValue=Config.DefaultMaxSpl, TunabilityNumber=1, MinValue=[], MaxValue=[], BankNumber=0, PreOverlay=false, PostOverlay=false, UseSameName=on}
      mask prompts: TriggerInit "Hidden: MoveFcn redraw"; TopName "Name:"; TuneName "Name of TuneVar:"; DataTypeOut "Data type:"; MaskValue "Default Value:"; TunabilityNumber "Tunability:"; MinValue "Min Value:"; MaxValue "Max Value:"; BankNumber "Target memory bank number:"; PreOverlay "Requires pre-overlay action:"; PostOverlay "Requires post-overlay action:"; UseSameName "Use same name for tune variable and TOP"
      mask help: The TuneTOP block encapsultes a Target Overlay Parameter, a Tune Variable, and a Trivial Translation between them.
      mask init:
      | [ok,activeTopPath,activeTunePath] = TuneTOP_Mask.Init(gcbh);
      settings: MoveFcn=TuneTOP_Mask.CB_TriggerInit(gcbh);
      mask Callback TriggerInit: TuneTOP_Mask.CB_TriggerInit(gcbh);
      mask TypeOptions TopName: TOP/TopName
      mask TypeOptions TuneName: Tune Variable/TuneName
      mask TypeOptions DataTypeOut: TOP/DataTypeOut
      mask TypeOptions MaskValue: Tune Variable/MaskValue
      mask TypeOptions TunabilityNumber: Tune Variable/TunabilityNumber
      mask Callback TunabilityNumber: TuneVarMask.CB_TunabilityNumber(gcbh);
      mask TypeOptions MinValue: Tune Variable/MinValue
      mask TypeOptions MaxValue: Tune Variable/MaxValue
      mask TypeOptions BankNumber: TOP/BankNumber
      mask TypeOptions PreOverlay: TOP/PreOverlay
      mask TypeOptions PostOverlay: TOP/PostOverlay
      mask Callback UseSameName: TuneTOP_Mask.CB_UseSameName(gcbh);
      mask DialogControl toolPanel Prompt: Tuning Tool Hints
      mask DialogControl DescriptionGroup Prompt: Description
      mask DialogControl EditDescription Prompt: Edit Description
      mask DialogControl EditDescription Callback: TuneTOP_Mask.CB_EditDescription(gcbh);
      mask DialogControl TunabilityText Prompt: Easy: Changes nearly every tuning.
      mask DialogControl AdvancedPanel Prompt: Advanced
      mask DialogControl ConvertToFullTranslation Prompt: Irreversible conversion to full translation
      mask DialogControl ConvertToFullTranslation Callback: TuneTOP_Mask.CB_ConvertToFullTranslation(gcbh);
      mask DialogControl ErrorContainer Prompt: Error Messages
      mask Display:
      | % retrieve icon definition
      | [path,w,h] = TuneTOP_Mask.Icon();
      | 
      | % retrieve the block's pixel size
      | pos = get(gcbh,'position');
      | bw = pos(3) - pos(1);
      | bh = pos(4) - pos(2);
      | 
      | % draw centered icon
      | xAdj = bw/2 - w/2 + 5;
      | yAdj = bh/2 - h/2 + 4;
      | for i=1:length(path)
      | 	patch(path(i).x+xAdj, path(i).y+yAdj, path(i).rgb);
      | end
      | 
      | % show the top name or an X
      | if (exist('ok','var') && ok)
      | 	text(bw*0.5, bh*0.2, activeTopPath, 'horizontalAlignment', 'center');
      | 	patch(0,0,[1 1 1]);
      | 	patch(bw,bh,[1 1 1]);
      | else
      | 	tx=bw*0.03;
      | 	ty=bh*0.03;
      | 	patch([0 tx bw bw-tx], [ty 0 bh-ty bh], [1 0 0]);
      | 	patch([0 bw-tx bw tx], [bh-ty 0 ty bh], [1 0 0]);
      | end

== system Model_TranslationEngine64/NEAR/Near1p1/VolumeMute/VolMuteCh2/Ann2NonEntVncApplied/nonentVNCApplied_subsystem ==
  TuneTOP : Subsystem
